simulink model "z2"  (R2017b)
settings: Solver=FixedStepDiscrete  StartTime=0.0  StopTime=0  RelTol=1e-3
libraries: CPOiS_SourcesSinks x9, CPOiS_DataManipulation x3, CPOiS_HistogramOperations x2
settings Model: Creator=alis  LastModifiedBy=alis

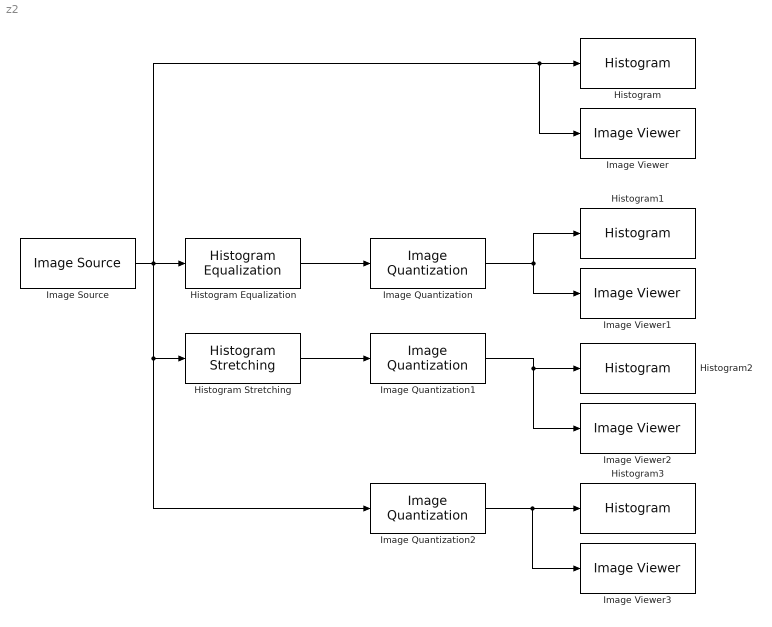
== system z2 ==
  Histogram{,1..3} (4 alike) : CPOiS_SourcesSinks/Histogram
      settings: SourceProductName=CPOiS - Digital image and signal processing
  Histogram Equalization : CPOiS_HistogramOperations/Histogram Equalization
      settings: SourceProductName=CPOiS - Digital image and signal processing
  Histogram Stretching : CPOiS_HistogramOperations/Histogram Stretching
      settings: SourceProductName=CPOiS - Digital image and signal processing
  Image Quantization : CPOiS_DataManipulation/Image Quantization  LevelsNum=8
      settings: SourceProductName=CPOiS - Digital image and signal processing
  Image Quantization1 : CPOiS_DataManipulation/Image Quantization  LevelsNum=8
      settings: SourceProductName=CPOiS - Digital image and signal processing
  Image Quantization2 : CPOiS_DataManipulation/Image Quantization  LevelsNum=8
      settings: SourceProductName=CPOiS - Digital image and signal processing
  Image Source : CPOiS_SourcesSinks/Image Source  FileSelection=foggyroad.jpg
      settings: SourceProductName=CPOiS - Digital image and signal processing
  Image Viewer{,1..3} (4 alike) : CPOiS_SourcesSinks/Image Viewer
      settings: SourceProductName=CPOiS - Digital image and signal processing
  wires:
  Histogram Equalization/1 -> Image Quantization/1
  Image Source/1 -> Image Viewer/1, Histogram/1, Image Quantization2/1, Histogram Stretching/1, Histogram Equalization/1
  Histogram Stretching/1 -> Image Quantization1/1
  Image Quantization/1 -> Image Viewer1/1, Histogram1/1
  Image Quantization1/1 -> Image Viewer2/1, Histogram2/1
  Image Quantization2/1 -> Image Viewer3/1, Histogram3/1
